simulink model "schema_fig18"  (R2023b)
settings: Solver=VariableStepAuto  StartTime=0.0  StopTime=100  RelTol=1e-3
settings Model: Creator=Daniela  LastModifiedBy=Daniela

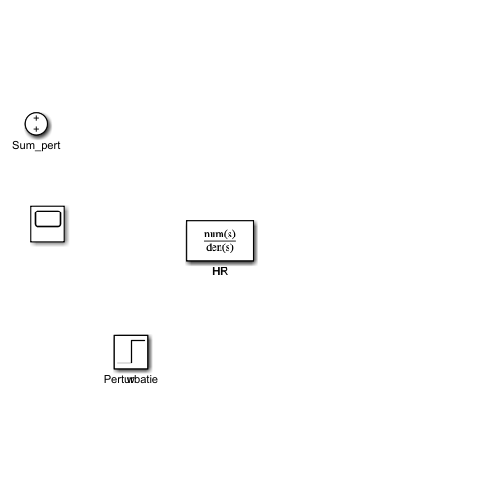
[thumbnail: Simulink's stored preview of the top-level diagram]
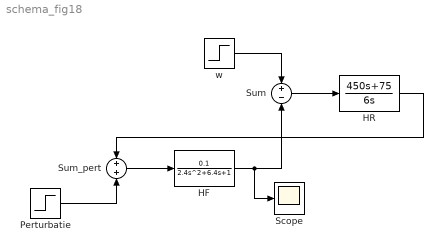
== system schema_fig18 ==
  HF : TransferFcn  Numerator=0.1  Denominator=[2.4 6.4 1]
  HR : TransferFcn  Numerator=[450 75]  Denominator=[6 0]
  Perturbatie : Step  Time=0  After=0  SampleTime=0
  Scope : Scope
  Sum : Sum  Inputs=+-
  Sum_pert : Sum
  w : Step  Time=0  SampleTime=0
  wires:
  w/1 -> Sum/1
  Perturbatie/1 -> Sum_pert/2
  Sum_pert/1 -> HF/1
  HF/1 -> Sum/2, Scope/1
  Sum/1 -> HR/1
  HR/1 -> Sum_pert/1
